simulink model "Simulation"  (R2021b)
settings: Solver=VariableStepAuto  StartTime=0.0  StopTime=150  RelTol=1e-3
values from neighbouring files (symbols this model uses):
  Ad = sysd.A    [StateSpace.m]    (also in StateSpace.mat = [0.99194127447 -0.000254162269677 -6.42347193166e-06 0.00010)
  Bd = sysd.B    [StateSpace.m]    (also in StateSpace.mat = [1.49694994056  -0.00781482451497; 0.0111300854252  0.015539)
  Cd = sysd.C    [StateSpace.m]    (also in StateSpace.mat = [1 0 0 0 0 1 0 0 0 0 1 0 ... (16 elements, 4x4)])
  Dd = sysd.D    [StateSpace.m]    (also in StateSpace.mat = [0  0; 0  0; 0  0; 0  0])
  F = real(C * phi)    [StateSpace.m]    (also in StateSpace.mat = [-0.40486417466 0.00197426364685 -0.000887607233206 -0.00071)
  G = real(C * inv(A) * (phi-eye(4)) * B)    [StateSpace.m]    (also in StateSpace.mat = [584.762838811  4.65927843492; -2.71097312864  0.29525659877)
  Q = diag([0, 0, 1, 0])    [StateSpace.m]    (also in StateSpace.mat = [0 0 0 0 0 0 0 0 0 0 1 0 ... (16 elements, 4x4)])
  R = diag([0, 1])    [StateSpace.m]    (also in StateSpace.mat = [0  0; 0  1])
libraries: aerolibfltsims x1
settings Model: Creator=AbinayBrown  LastModifiedBy=AbinayBrown

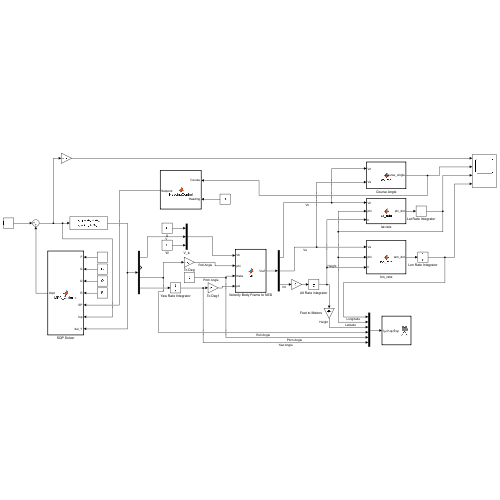
[thumbnail: Simulink's stored preview of the top-level diagram]
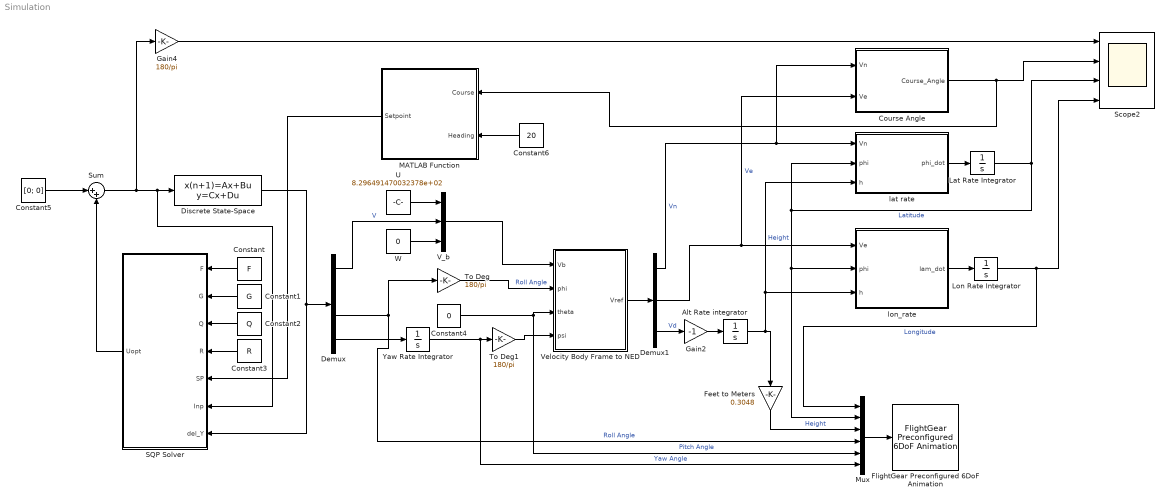
== system Simulation ==
  Alt Rate integrator : Integrator  InitialCondition=20000
  Constant : Constant  Value=F
  Constant1 : Constant  Value=G
  Constant2 : Constant  Value=Q
  Constant3 : Constant  Value=R
  Constant4 : Constant  Value=0
  Constant5 : Constant  Value=[0; 0]
  Constant6 : Constant  Value=20
  Course Angle : MATLAB Function  TreatAsAtomicUnit=on
  Demux : Demux
  Demux1 : Demux  Outputs=3
  Discrete State-Space : DiscreteStateSpace  A=Ad  B=Bd  C=Cd  D=Dd  InitialCondition=[0; 0; 0; 0];  SampleTime=0.1
  Feet to Meters : Gain  Gain=0.3048
  FlightGear Preconfigured 6DoF Animation : aerolibfltsims/FlightGear Preconfigured 6DoF Animation  xFlightGearVersion=v2019.1  DestinationIpAddress=127.0.0.1  DestinationPort=5502  SampleTime=1/30  packetVersion=24
  Gain2 : Gain  Gain=-1
  Gain4 : Gain  Gain=180/pi
  Lat Rate Integrator : Integrator  InitialCondition=40.683305
  Lon Rate Integrator : Integrator  InitialCondition=-74.074123
  MATLAB Function : MATLAB Function  TreatAsAtomicUnit=on
  Mux : Mux  Inputs=6
  SQP Solver : MATLAB Function  TreatAsAtomicUnit=on
  Scope2 : Scope  NumInputPorts=4
  Sum : Sum  Inputs=|++
  To Deg : Gain  Gain=180/pi
  To Deg1 : Gain  Gain=180/pi
  U : Constant  Value=8.296491470032378e+02
  V_b : Mux  Inputs=3
  Velocity Body Frame to NED : MATLAB Function  TreatAsAtomicUnit=on
  W : Constant  Value=0
  Yaw Rate Integrator : Integrator
  lat rate : MATLAB Function  TreatAsAtomicUnit=on
  lon_rate : MATLAB Function  TreatAsAtomicUnit=on
  wires:
  Discrete State-Space/1 -> SQP Solver/7(del_Y), Demux/1
  Constant/1 -> SQP Solver/1(F)
  Constant1/1 -> SQP Solver/2(G)
  Constant2/1 -> SQP Solver/3(Q)
  Constant3/1 -> SQP Solver/4(R)
  Constant5/1 -> Sum/1
  SQP Solver/1(Uopt) -> Sum/2
  Demux/4 -> Yaw Rate Integrator/1
  To Deg/1 -> Velocity Body Frame to NED/2(phi)  "Roll Angle"
  To Deg1/1 -> Velocity Body Frame to NED/4(psi)
  Demux/1 -> V_b/2  "V"
  Sum/1 -> Gain4/1, SQP Solver/6(Inp), Discrete State-Space/1
  U/1 -> V_b/1
  W/1 -> V_b/3
  V_b/1 -> Velocity Body Frame to NED/1(Vb)
  Velocity Body Frame to NED/1(Vref) -> Demux1/1
  Demux1/1 -> Course Angle/1(Vn), lat rate/1(Vn)  "Vn"
  Demux1/2 -> Course Angle/2(Ve), lon_rate/1(Ve)  "Ve"
  Demux/3 -> Mux/4, To Deg/1  "Roll Angle"
  Yaw Rate Integrator/1 -> Mux/6, To Deg1/1  "Yaw Angle"
  lat rate/1(phi_dot) -> Lat Rate Integrator/1
  Lat Rate Integrator/1 -> Scope2/3, Mux/2, lon_rate/2(phi), lat rate/2(phi)  "Latitude"
  Gain2/1 -> Alt Rate integrator/1
  Demux1/3 -> Gain2/1  "Vd"
  lon_rate/1(lam_dot) -> Lon Rate Integrator/1
  Lon Rate Integrator/1 -> Mux/1, Scope2/4  "Longitude"
  Constant4/1 -> Mux/5, Velocity Body Frame to NED/3(theta)  "Pitch Angle"
  Alt Rate integrator/1 -> Feet to Meters/1, lat rate/3(h), lon_rate/3(h)  "Height"
  Mux/1 -> FlightGear Preconfigured 6DoF Animation/1
  Gain4/1 -> Scope2/1
  Feet to Meters/1 -> Mux/3  "Height"
  Course Angle/1(Course_Angle) -> MATLAB Function/1(Course), Scope2/2
  MATLAB Function/1(Setpoint) -> SQP Solver/5(SP)
  Constant6/1 -> MATLAB Function/2(Heading)

== matlab function Simulation/Velocity Body Frame to NED ==
  data: Vb input; Vref output; phi input; theta input; psi input
function  Vref = fcn(Vb, phi, theta, psi)
    phi =   (pi/180) * phi;
    theta = (pi/180) * theta;
    psi =   (pi/180) * psi;
    Rot1 = [cos(psi), sin(psi), 0;
           -sin(psi), cos(psi), 0;
           0 , 0, 1];
    Rot2 = [cos(theta), 0, -sin(theta);
           0, 1, 0;
           sin(theta), 0, cos(theta)];
    Rot3 = [1, 0, 0;
           0, cos(phi), sin(phi);
           0, -sin(phi), cos(phi)];
    Vref = (Rot3*Rot2*Rot1)'*Vb;
end

== matlab function Simulation/SQP Solver ==
  data: F input; G input; Q input; R input; SP input; Inp input; del_Y input; Uopt output size=[2,1]
function Uopt = MPC_Optimize(F, G, Q, R, SP, Inp, del_Y)
    Uopt = zeros(2,1);
    coder.extrinsic('Optimize');
    Uopt = Optimize(F, G, Q, R, SP, Inp, del_Y);
end

== matlab function Simulation/Course Angle ==
  data: Vn input; Course_Angle output; Ve input
function  Course_Angle = course(Vn, Ve)
    Course_Angle = 90 - (180/pi)*atan2(Vn, Ve);
end

== matlab function Simulation/lat rate ==
  data: Vn input; phi_dot output; phi input; h input
function phi_dot = lat_rate(Vn, phi, h)
    phi = (pi/180)*phi;
    a = 20925646.33;
    e = 0.08181919084;
    M = a*(1-e^2)/((1-(e^2)*(sin(phi)^2))^1.5);
    phi_dot = (180/pi) * (Vn/(M+h));
end

== matlab function Simulation/lon_rate ==
  data: Ve input; lam_dot output; phi input; h input
function lam_dot = lon_rate(Ve, phi, h)
    phi = (pi/180)*phi;
    a = 20925646.33;
    e = 0.08181919084;
    N = a/((1-(e^2)*(sin(phi)^2))^1.5);
    lam_dot = (180/pi) * (Ve/(N+h)/cos(phi));
end

== matlab function Simulation/MATLAB Function ==
  data: Course input; Setpoint output; Heading input
function Setpoint = HeadingControl(Course, Heading)
    Error = (Heading - Course)/Heading;
    MaxBank = 25 * (pi/180);
    if abs(Error) < 0.2
        Setpoint = MaxBank * Error;
    else 
        Setpoint = MaxBank;
    end
end
